simulink model "BPAM_Shell"  (R2015a)
settings: Solver=FixedStepDiscrete  SolverMode=SingleTasking  StartTime=0.0  StopTime=(12+256+8+602+4)*8  RelTol=1e-3
undefined symbols (not defined in the file or in its folder): K1t, K2t, rcosine
libraries: simulink x2
settings Model: Creator=Jensen  LastModifiedBy=ecenstudent
settings DebuggingCC: UnderspecifiedInitializationDetection=Classic  MergeDetectMultiDrivingBlocksExec=none  SolverPrmCheckMsg=warning  StateNameClashWarn=warning

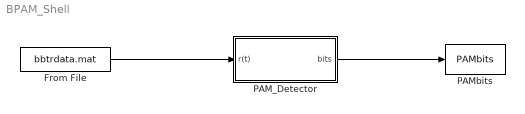
== system BPAM_Shell ==
  From File : FromFile  FileName=bbtrdata.mat  SampleTime=1
  PAM_Detector : Subsystem
  PAMbits : ToWorkspace  VariableName=PAMbits  SampleTime=-1
      settings: Decimation=2
  wires:
  PAM_Detector/1(bits) -> PAMbits/1
  From File/1 -> PAM_Detector/1(r(t))

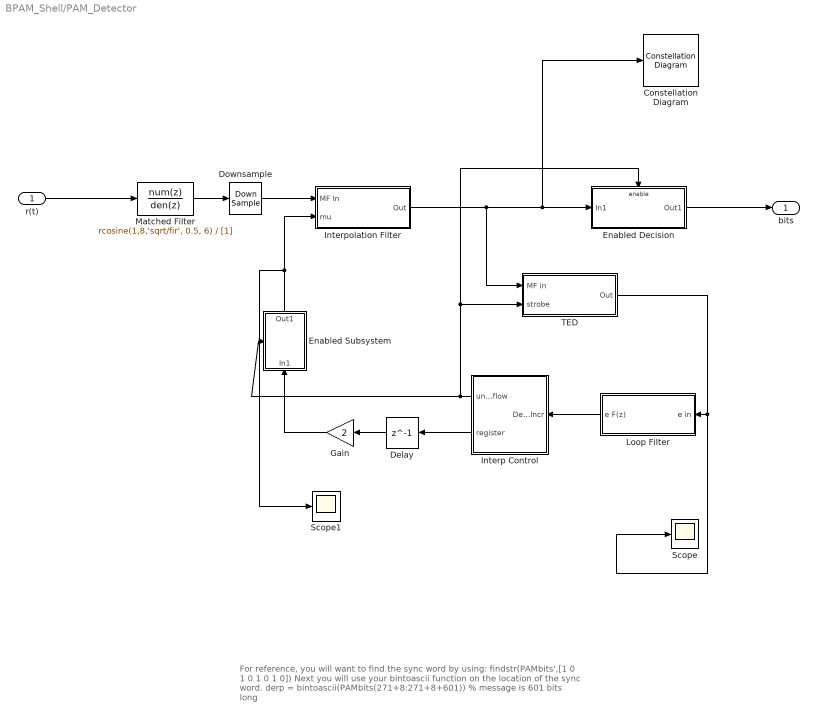
== system BPAM_Shell/PAM_Detector ==
  note: For reference, you will want to find the sync word by using:
      |
      | findstr(PAMbits',[1 0 1 0 1 0 1 0])
      |
      | Next you will use your bintoascii function on the location of the sync word.
      |
      | derp = bintoascii(PAMbits(271+8:271+8+601)) % message is 601 bits  long
  r(t) : Inport
  Constellation Diagram : ConstellationDiagram
  Delay : Delay  DelayLength=1
  Downsample : DownSample  N=4  phase=1  InputProcessing=Inherited (this choice will be removed - see release notes)
  Enabled Decision : Subsystem  TreatAsAtomicUnit=on
  Enabled Subsystem : Subsystem  TreatAsAtomicUnit=on
  Gain : Gain  Gain=2
  Interp Control : Subsystem
  Interpolation Filter : Subsystem
  Loop Filter : Subsystem
  Matched Filter : DiscreteFilter  Numerator=rcosine(1,8,'sqrt/fir', 0.5, 6)  Denominator=[1]  SampleTime=1
  Scope : Scope
      settings: YMin=-0.98467  YMax=1.4536
  Scope1 : Scope
      settings: YMin=-0.125  YMax=1.125
  TED : Subsystem
  bits : Outport
  wires:
  Matched Filter/1 -> Downsample/1
  r(t)/1 -> Matched Filter/1
  Downsample/1 -> Interpolation Filter/1(MF In)
  Interpolation Filter/1(Out) -> TED/1(MF in), Constellation Diagram/1, Enabled Decision/1(In1)
  Enabled Subsystem/1(Out1) -> Interpolation Filter/2(mu), Scope1/1
  Delay/1 -> Gain/1
  Gain/1 -> Enabled Subsystem/1(In1)
  Interp Control/2(register) -> Delay/1
  Loop Filter/1(e F(z)) -> Interp Control/1(Delta Incr)
  Interp Control/1(underflow) -> Enabled Subsystem/Enable, TED/2(strobe), Enabled Decision/Enable
  TED/1(Out) -> Scope/1, Loop Filter/1(e in)
  Enabled Decision/1(Out1) -> bits/1

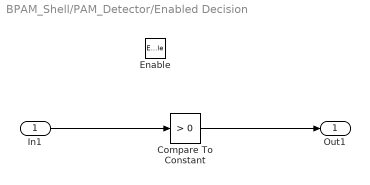
== system BPAM_Shell/PAM_Detector/Enabled Decision ==
  In1 : Inport
  Enable : EnablePort
  Compare To Constant : simulink/Logic and Bit Operations/Compare To Constant  relop=>  const=0  OutDataTypeStr=boolean
  Out1 : Outport
  wires:
  In1/1 -> Compare To Constant/1
  Compare To Constant/1 -> Out1/1

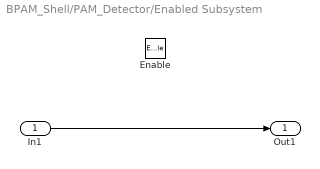
== system BPAM_Shell/PAM_Detector/Enabled Subsystem ==
  In1 : Inport
  Enable : EnablePort
  Out1 : Outport
  wires:
  In1/1 -> Out1/1

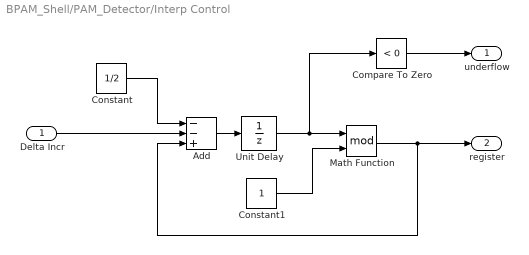
== system BPAM_Shell/PAM_Detector/Interp Control ==
  Delta Incr : Inport
  Add : Sum  Inputs=--+
  Compare To Zero : simulink/Logic and Bit Operations/Compare To Zero  relop=<  OutDataTypeStr=boolean
  Constant : Constant  Value=1/2
  Constant1 : Constant
  Math Function : Math  Operator=mod  SaturateOnIntegerOverflow=on
  Unit Delay : UnitDelay  SampleTime=-1
  underflow : Outport
  register : Outport  Port=2
  wires:
  Delta Incr/1 -> Add/2
  Constant/1 -> Add/1
  Add/1 -> Unit Delay/1
  Constant1/1 -> Math Function/2
  Unit Delay/1 -> Compare To Zero/1, Math Function/1
  Math Function/1 -> Add/3, register/1
  Compare To Zero/1 -> underflow/1

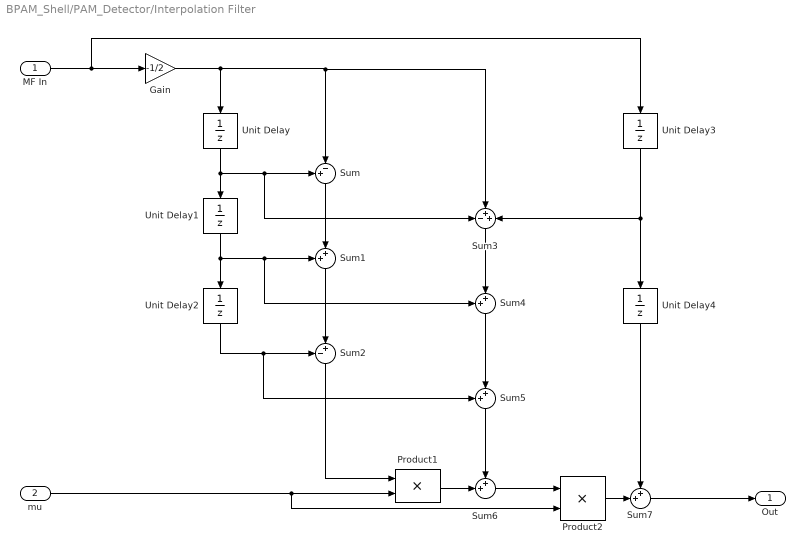
== system BPAM_Shell/PAM_Detector/Interpolation Filter ==
  MF In : Inport
  mu : Inport  Port=2
  Gain : Gain  Gain=-1/2
  Product1 : Product  SaturateOnIntegerOverflow=on  InputSameDT=on  OutDataTypeStr=Inherit: Same as first input
  Product2 : Product  SaturateOnIntegerOverflow=on  InputSameDT=on  OutDataTypeStr=Inherit: Same as first input
  Sum : Sum  Inputs=+-|  SaturateOnIntegerOverflow=on  InputSameDT=on  OutDataTypeStr=Inherit: Same as first input
  Sum{1,4..7} (5 alike) : Sum  Inputs=++|  SaturateOnIntegerOverflow=on  InputSameDT=on  OutDataTypeStr=Inherit: Same as first input
  Sum2 : Sum  Inputs=-+|  SaturateOnIntegerOverflow=on  InputSameDT=on  OutDataTypeStr=Inherit: Same as first input
  Sum3 : Sum  Inputs=-++  SaturateOnIntegerOverflow=on  InputSameDT=on  OutDataTypeStr=Inherit: Same as first input
  Unit Delay{,1..4} (5 alike) : UnitDelay  SampleTime=-1
  Out : Outport
  wires:
  Sum1/1 -> Sum2/2
  Sum/1 -> Sum1/2
  Unit Delay/1 -> Sum3/1, Sum/1, Unit Delay1/1
  Unit Delay1/1 -> Sum4/1, Sum1/1, Unit Delay2/1
  Unit Delay2/1 -> Sum5/1, Sum2/1
  Sum5/1 -> Sum6/1
  Product1/1 -> Sum6/2
  Sum4/1 -> Sum5/2
  Sum3/1 -> Sum4/2
  MF In/1 -> Unit Delay3/1, Gain/1
  Gain/1 -> Unit Delay/1, Sum/2, Sum3/2
  Product2/1 -> Sum7/2
  Unit Delay4/1 -> Sum7/1
  Sum6/1 -> Product2/1
  Sum7/1 -> Out/1
  Unit Delay3/1 -> Sum3/3, Unit Delay4/1
  Sum2/1 -> Product1/1
  mu/1 -> Product2/2, Product1/2

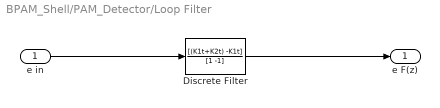
== system BPAM_Shell/PAM_Detector/Loop Filter ==
  e in : Inport
  Discrete Filter : DiscreteFilter  Numerator=[(K1t+K2t) -K1t]  Denominator=[1 -1]
  e F(z) : Outport
  wires:
  e in/1 -> Discrete Filter/1
  Discrete Filter/1 -> e F(z)/1

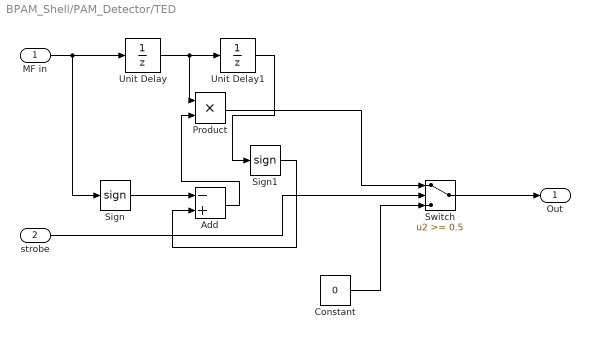
== system BPAM_Shell/PAM_Detector/TED ==
  MF in : Inport
  strobe : Inport  Port=2
  Add : Sum  Inputs=-+
  Constant : Constant  Value=0
  Product : Product
  Sign : Signum
  Sign1 : Signum
  Switch : Switch  Threshold=0.5  SaturateOnIntegerOverflow=on
  Unit Delay : UnitDelay  SampleTime=-1
  Unit Delay1 : UnitDelay  SampleTime=-1
  Out : Outport
  wires:
  Switch/1 -> Out/1
  Constant/1 -> Switch/3
  strobe/1 -> Switch/2
  MF in/1 -> Sign/1, Unit Delay/1
  Unit Delay/1 -> Product/1, Unit Delay1/1
  Sign/1 -> Add/1
  Add/1 -> Product/2
  Unit Delay1/1 -> Sign1/1
  Sign1/1 -> Add/2
  Product/1 -> Switch/1
